simulink model "sim_line_seg_ctrl_with_pi_ctrl"  (R2021b)
settings: Solver=ode1  StartTime=0.0  StopTime=inf  FixedStep=0.01  RelTol=1e-3
libraries: slpidlib x2, mobileRoboticsLib x1
settings Model: Creator=ASUS  LastModifiedBy=ASUS

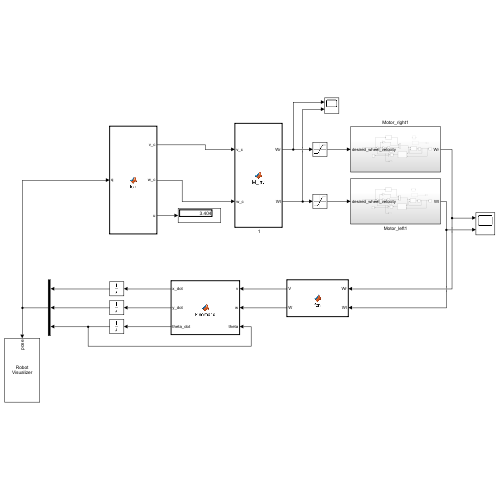
[thumbnail: Simulink's stored preview of the top-level diagram]
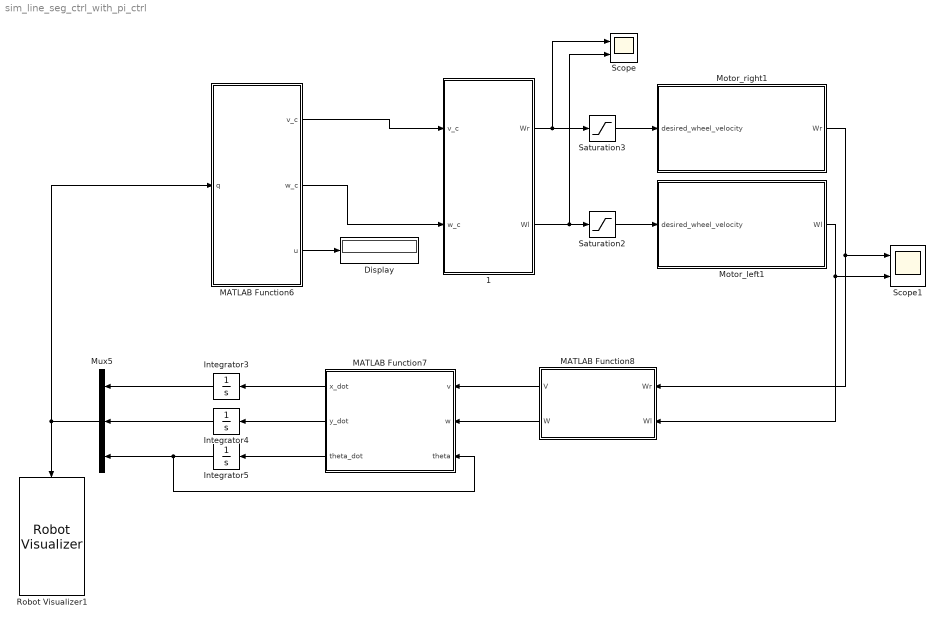
== system sim_line_seg_ctrl_with_pi_ctrl ==
  " 1" : MATLAB Function  TreatAsAtomicUnit=on
  Display : Display
  Integrator3 : Integrator  InitialCondition=5
  Integrator4 : Integrator  InitialCondition=1
  Integrator5 : Integrator  InitialCondition=0.6*pi
  MATLAB Function6 : MATLAB Function  TreatAsAtomicUnit=on
  MATLAB Function7 : MATLAB Function  TreatAsAtomicUnit=on
  MATLAB Function8 : MATLAB Function  TreatAsAtomicUnit=on
  Motor_left1 : Subsystem
  Motor_right1 : Subsystem
  Mux5 : Mux  Inputs=3
  Robot Visualizer1 : mobileRoboticsLib/Environments/Robot Visualizer  robotRadius=0.44  showTrajectory=on  hasWaypoints=off  hasLidar=off  sensorOffset=[ 0, 0 ]  scanAngles=[ -pi/4, 0, pi/4 ]  hasObjDetector=off  objDetectorOffset=[ 0, 0 ]  objDetectorAngle=0  objDetectorFOV=pi/4  objDetectorMaxRange=5  objectColors=[ 1, 0, 0; 0, 1, 0; 0, 0, 1 ]  objectMarkers=s
  Saturation2 : Saturate  UpperLimit=14  LowerLimit=-14
  Saturation3 : Saturate  UpperLimit=14  LowerLimit=-14
  Scope : Scope  NumInputPorts=2
  Scope1 : Scope  NumInputPorts=2
  wires:
  MATLAB Function7/2(y_dot) -> Integrator4/1
  Integrator5/1 -> Mux5/3, MATLAB Function7/3(theta)
  Integrator4/1 -> Mux5/2
  MATLAB Function8/1(V) -> MATLAB Function7/1(v)
  Integrator3/1 -> Mux5/1
  MATLAB Function8/2(W) -> MATLAB Function7/2(w)
  Mux5/1 -> Robot Visualizer1/1, MATLAB Function6/1(q)
  MATLAB Function7/1(x_dot) -> Integrator3/1
  MATLAB Function7/3(theta_dot) -> Integrator5/1
  MATLAB Function6/1(v_c) -> " 1"/1(v_c)
  MATLAB Function6/2(w_c) -> " 1"/2(w_c)
  " 1"/1(Wr) -> Scope/1, Saturation3/1
  Saturation3/1 -> Motor_right1/1(desired_wheel_velocity)
  " 1"/2(Wl) -> Scope/2, Saturation2/1
  Saturation2/1 -> Motor_left1/1(desired_wheel_velocity)
  Motor_right1/1(Wr) -> MATLAB Function8/1(Wr), Scope1/1
  Motor_left1/1(Wl) -> MATLAB Function8/2(Wl), Scope1/2
  MATLAB Function6/3(u) -> Display/1

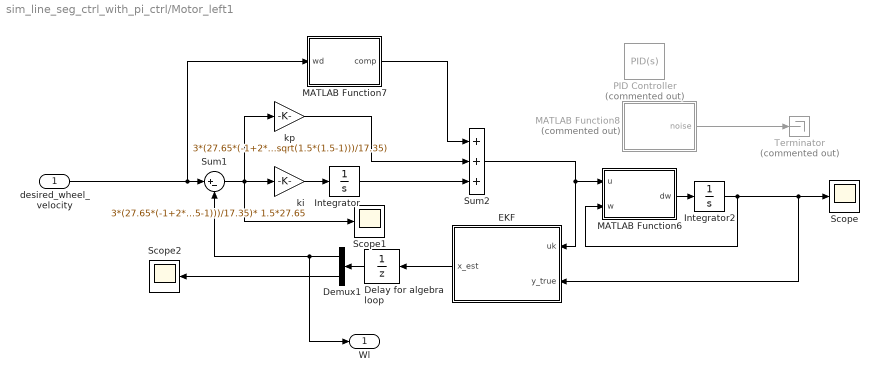
== system sim_line_seg_ctrl_with_pi_ctrl/Motor_left1 ==
  desired_wheel_velocity : Inport
  Delay for algebra loop : UnitDelay  SampleTime=-1  HasFrameUpgradeWarning=on
  Demux1 : Demux  Outputs=[1,3]
  EKF : MATLAB Function  TreatAsAtomicUnit=on
  Integrator : Integrator
  Integrator2 : Integrator
  MATLAB Function6 : MATLAB Function  TreatAsAtomicUnit=on
  MATLAB Function7 : MATLAB Function  TreatAsAtomicUnit=on
  MATLAB Function8 : MATLAB Function  Commented=on  TreatAsAtomicUnit=on
  PID Controller : slpidlib/PID Controller  Commented=on  Controller=PID  Form=Parallel  TimeDomain=Continuous-time  UseExternalTs=off  SampleTime=-1  IntegratorMethod=Forward Euler  FilterMethod=Forward Euler  ControllerParametersSource=internal  P=3*(27.65*(-1+2*1.5-2*sqrt(1.5*(1.5-1)))/17.35)  I=3*(27.65*(-1+2*1.5-2*sqrt(1.5*(1.5-1)))/17.35)* 1.5*27.65  D=0  UseFilter=on  N=100  TunerSelectOption=Transfer Function Based (PID Tuner App)  InitialConditionSource=internal  InitialConditionForIntegrator=0  InitialConditionForFilter=0  DifferentiatorICPrevScaledInput=0  ExternalReset=none  TrackingMode=off  Kt=1  LimitOutput=off  SatLimitsSource=internal  UpperSaturationLimit=inf  LowerSaturationLimit=-inf  LinearizeAsGain=on  AntiWindupMode=none  Kb=1  POutMin=[]  POutMax=[]  IOutMin=[]  IOutMax=[]  DOutMin=[]  DOutMax=[]  NOutMin=[]  NOutMax=[]  SumOutMin=[]  SumOutMax=[]  SaturationOutMin=[]  SaturationOutMax=[]  PParamMin=[]  PParamMax=[]  IParamMin=[]  IParamMax=[]  DParamMin=[]  DParamMax=[]  NParamMin=[]  NParamMax=[]  KbParamMin=[]  KbParamMax=[]  KtParamMin=[]  KtParamMax=[]  KbOutMin=[]  KbOutMax=[]  KtOutMin=[]  KtOutMax=[]  IntegratorOutMin=[]  IntegratorOutMax=[]  FilterOutMin=[]  FilterOutMax=[]  SumI1OutMin=[]  SumI1OutMax=[]  SumI2OutMin=[]  SumI2OutMax=[]  SumI3OutMin=[]  SumI3OutMax=[]  SumI4OutMin=[]  SumI4OutMax=[]  SumDOutMin=[]  SumDOutMax=[]  DifferentiatorOutMin=[]  DifferentiatorOutMax=[]  FilterDiffOutCoefMin=[]  FilterDiffOutCoefMax=[]  ReciprocalOutMin=[]  ReciprocalOutMax=[]  SumDenOutMin=[]  SumDenOutMax=[]  SumNumOutMin=[]  SumNumOutMax=[]  DivideOutMin=[]  DivideOutMax=[]  UdiffTsProdOutMin=[]  UdiffTsProdOutMax=[]  NTsProdOutMin=[]  NTsProdOutMax=[]  UintegralTsProdOutMin=[]  UintegralTsProdOutMax=[]  UngainTsProdOutMin=[]  UngainTsProdOutMax=[]  IntegratorContinuousStateAttributes=''  IntegratorStateMustResolveToSignalObject=off  IntegratorRTWStateStorageClass=Auto  FilterContinuousStateAttributes=''  FilterStateMustResolveToSignalObject=off  FilterRTWStateStorageClass=Auto  ParallelPVariant=InternalParameters  IdealPVariant=Disabled  IVariant=InternalParameters  DVariant=InternalParameters  IntegratorVariant=Continuous  SatVariant=Disabled  AWVariant=Passthrough  PCopyVariant=Disabled  TRVariant=Disabled  FdbkBlocksVariant=Forward  IdealPFdbkVariant=Disabled  SatFdbkVariant=Disabled  DerivativeFilterVariant=ContFilter  NVariant=InternalParameters  NCopyVariant=Disabled  FilterICVariant=InternalICsFilter  IntegratorICVariant=InternalICs  ExternalResetVariant=Disabled  TRSumVariant=Passthrough  SumFdbkVariant=Disabled  SumVariant=Sum_PID  TsampFilterVariant=InternalTs  TsampNgainVariant=Passthrough  TsampIntegralVariant=Passthrough  ExternalSaturationOutDataTypeStr=Inherit: Same as second input
  Scope : Scope
  Scope1 : Scope
  Scope2 : Scope
  Sum1 : Sum  Inputs=|+-
  Sum2 : Sum  Inputs=+++
  Terminator : Terminator  Commented=on
  ki : Gain  Gain=3*(27.65*(-1+2*1.5-2*sqrt(1.5*(1.5-1)))/17.35)* 1.5*27.65
  kp : Gain  Gain=3*(27.65*(-1+2*1.5-2*sqrt(1.5*(1.5-1)))/17.35)
  Wl : Outport
  wires:
  Sum2/1 -> MATLAB Function6/1(u), EKF/1(uk)
  MATLAB Function6/1(dw) -> Integrator2/1
  Integrator/1 -> Sum2/3
  kp/1 -> Sum2/2
  MATLAB Function7/1(comp) -> Sum2/1
  Demux1/1 -> Wl/1, Sum1/2
  Delay for algebra loop/1 -> Demux1/1
  desired_wheel_velocity/1 -> MATLAB Function7/1(wd), Sum1/1
  Sum1/1 -> ki/1, Scope1/1, kp/1
  ki/1 -> Integrator/1
  Demux1/2 -> Scope2/1
  MATLAB Function8/1(noise) -> Terminator/1
  Integrator2/1 -> MATLAB Function6/2(w), Scope/1, EKF/2(y_true)
  EKF/1(x_est) -> Delay for algebra loop/1

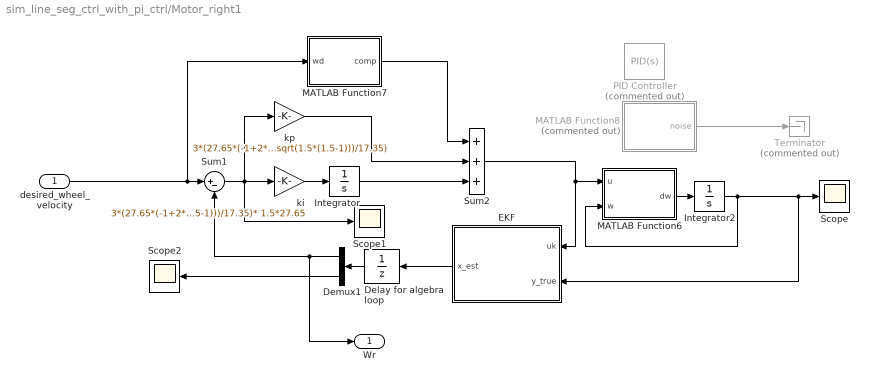
== system sim_line_seg_ctrl_with_pi_ctrl/Motor_right1 ==
  desired_wheel_velocity : Inport
  Delay for algebra loop : UnitDelay  SampleTime=-1  HasFrameUpgradeWarning=on
  Demux1 : Demux  Outputs=[1,3]
  EKF : MATLAB Function  TreatAsAtomicUnit=on
  Integrator : Integrator
  Integrator2 : Integrator
  MATLAB Function6 : MATLAB Function  TreatAsAtomicUnit=on
  MATLAB Function7 : MATLAB Function  TreatAsAtomicUnit=on
  MATLAB Function8 : MATLAB Function  Commented=on  TreatAsAtomicUnit=on
  PID Controller : slpidlib/PID Controller  Commented=on  Controller=PID  Form=Parallel  TimeDomain=Continuous-time  UseExternalTs=off  SampleTime=-1  IntegratorMethod=Forward Euler  FilterMethod=Forward Euler  ControllerParametersSource=internal  P=3*(27.65*(-1+2*1.5-2*sqrt(1.5*(1.5-1)))/17.35)  I=3*(27.65*(-1+2*1.5-2*sqrt(1.5*(1.5-1)))/17.35)* 1.5*27.65  D=0  UseFilter=on  N=100  TunerSelectOption=Transfer Function Based (PID Tuner App)  InitialConditionSource=internal  InitialConditionForIntegrator=0  InitialConditionForFilter=0  DifferentiatorICPrevScaledInput=0  ExternalReset=none  TrackingMode=off  Kt=1  LimitOutput=off  SatLimitsSource=internal  UpperSaturationLimit=inf  LowerSaturationLimit=-inf  LinearizeAsGain=on  AntiWindupMode=none  Kb=1  POutMin=[]  POutMax=[]  IOutMin=[]  IOutMax=[]  DOutMin=[]  DOutMax=[]  NOutMin=[]  NOutMax=[]  SumOutMin=[]  SumOutMax=[]  SaturationOutMin=[]  SaturationOutMax=[]  PParamMin=[]  PParamMax=[]  IParamMin=[]  IParamMax=[]  DParamMin=[]  DParamMax=[]  NParamMin=[]  NParamMax=[]  KbParamMin=[]  KbParamMax=[]  KtParamMin=[]  KtParamMax=[]  KbOutMin=[]  KbOutMax=[]  KtOutMin=[]  KtOutMax=[]  IntegratorOutMin=[]  IntegratorOutMax=[]  FilterOutMin=[]  FilterOutMax=[]  SumI1OutMin=[]  SumI1OutMax=[]  SumI2OutMin=[]  SumI2OutMax=[]  SumI3OutMin=[]  SumI3OutMax=[]  SumI4OutMin=[]  SumI4OutMax=[]  SumDOutMin=[]  SumDOutMax=[]  DifferentiatorOutMin=[]  DifferentiatorOutMax=[]  FilterDiffOutCoefMin=[]  FilterDiffOutCoefMax=[]  ReciprocalOutMin=[]  ReciprocalOutMax=[]  SumDenOutMin=[]  SumDenOutMax=[]  SumNumOutMin=[]  SumNumOutMax=[]  DivideOutMin=[]  DivideOutMax=[]  UdiffTsProdOutMin=[]  UdiffTsProdOutMax=[]  NTsProdOutMin=[]  NTsProdOutMax=[]  UintegralTsProdOutMin=[]  UintegralTsProdOutMax=[]  UngainTsProdOutMin=[]  UngainTsProdOutMax=[]  IntegratorContinuousStateAttributes=''  IntegratorStateMustResolveToSignalObject=off  IntegratorRTWStateStorageClass=Auto  FilterContinuousStateAttributes=''  FilterStateMustResolveToSignalObject=off  FilterRTWStateStorageClass=Auto  ParallelPVariant=InternalParameters  IdealPVariant=Disabled  IVariant=InternalParameters  DVariant=InternalParameters  IntegratorVariant=Continuous  SatVariant=Disabled  AWVariant=Passthrough  PCopyVariant=Disabled  TRVariant=Disabled  FdbkBlocksVariant=Forward  IdealPFdbkVariant=Disabled  SatFdbkVariant=Disabled  DerivativeFilterVariant=ContFilter  NVariant=InternalParameters  NCopyVariant=Disabled  FilterICVariant=InternalICsFilter  IntegratorICVariant=InternalICs  ExternalResetVariant=Disabled  TRSumVariant=Passthrough  SumFdbkVariant=Disabled  SumVariant=Sum_PID  TsampFilterVariant=InternalTs  TsampNgainVariant=Passthrough  TsampIntegralVariant=Passthrough  ExternalSaturationOutDataTypeStr=Inherit: Same as second input
  Scope : Scope
  Scope1 : Scope
  Scope2 : Scope
  Sum1 : Sum  Inputs=|+-
  Sum2 : Sum  Inputs=+++
  Terminator : Terminator  Commented=on
  ki : Gain  Gain=3*(27.65*(-1+2*1.5-2*sqrt(1.5*(1.5-1)))/17.35)* 1.5*27.65
  kp : Gain  Gain=3*(27.65*(-1+2*1.5-2*sqrt(1.5*(1.5-1)))/17.35)
  Wr : Outport
  wires:
  Sum2/1 -> MATLAB Function6/1(u), EKF/1(uk)
  desired_wheel_velocity/1 -> MATLAB Function7/1(wd), Sum1/1
  Sum1/1 -> ki/1, Scope1/1, kp/1
  kp/1 -> Sum2/2
  MATLAB Function6/1(dw) -> Integrator2/1
  EKF/1(x_est) -> Delay for algebra loop/1
  MATLAB Function8/1(noise) -> Terminator/1
  Demux1/2 -> Scope2/1
  MATLAB Function7/1(comp) -> Sum2/1
  Integrator2/1 -> MATLAB Function6/2(w), EKF/2(y_true), Scope/1
  Demux1/1 -> Wr/1, Sum1/2
  Delay for algebra loop/1 -> Demux1/1
  ki/1 -> Integrator/1
  Integrator/1 -> Sum2/3

== matlab function sim_line_seg_ctrl_with_pi_ctrl/Motor_right1/MATLAB Function7 ==
  settings: updateMethod=DISCRETE
  data: wd input; comp output
function comp = fcn(wd)

b = 17.35 + rand; c = 5.63 + 0.3*rand;
comp = c/b*sign(wd);

== matlab function sim_line_seg_ctrl_with_pi_ctrl/Motor_right1/MATLAB Function8 ==
  data: noise output
function noise = fcn

noise = 0.1*randn;

== matlab function sim_line_seg_ctrl_with_pi_ctrl/MATLAB Function6 ==
  settings: updateMethod=DISCRETE
  data: q input; v_c output; w_c output; u output
function [v_c,w_c,u] = fcn(q)

T = [3, 0; 6, 4; 3, 4; 3, 1; 0, 3].';

persistent i
if isempty(i)
    i = 1;
end

if i>4
    i = 4;
end

dx = T(1,i+1) - T(1,i);
dy = T(2,i+1) - T(2,i);

v = [dx; dy]; 
vN = [dy; -dx];
r = q(1:2) - T(:,i);
u = v.'*r/(v.'*v);
if u>1
    i = i+1;
end
dn = vN.'*r/(vN.'*vN); % Normalized orthogonal distance
phiLin = atan2(v(2), v(1));
phiRot = atan(5*dn);
phiRef = wrapToPi(phiLin + phiRot);

ePhi = wrapToPi(phiRef - q(3));

v_c = 0.8*cos(ePhi);
w_c = 3*ePhi;

== matlab function sim_line_seg_ctrl_with_pi_ctrl/ 1 ==
  data: v_c input; Wr output; w_c input; Wl output
function [Wr, Wl] = M_inv(v_c, w_c)
r = 0.07;      %wheel radius
b = 0.22;      %length from wheel to wheel

Wr = ((2*v_c)+(w_c*b))/(2*r);
Wl = ((2*v_c)-(w_c*b))/(2*r);

== matlab function sim_line_seg_ctrl_with_pi_ctrl/MATLAB Function7 ==
  data: v input; x_dot output; w input; y_dot output; theta_dot output; theta input
function [x_dot,y_dot,theta_dot]= kinematic(v,w,theta)
x_dot = v*cos(theta);
y_dot = v*sin(theta);
theta_dot = w;

== matlab function sim_line_seg_ctrl_with_pi_ctrl/MATLAB Function8 ==
  data: Wr input; V output; Wl input; W output
function [V,W]= fcn(Wr,Wl)
r = 0.07;      %wheel radius
b = 0.22;      %length from wheel to wheel

V = r*(Wr/2) + r*(Wl/2);
W = r*(Wr/b) - r*(Wl/b);

== matlab function sim_line_seg_ctrl_with_pi_ctrl/Motor_left1/EKF ==
  settings: updateMethod=DISCRETE
  data: uk input; y_true input; x_est output
function x_est = EKF(uk,y_true)
Ts=0.01;
persistent x_est_p P Qd_est R_est Qc_est;
if isempty(x_est_p)
    
    x_est_p=[2;13;25;1];
    P=2*eye(4);
    Qc_est=1e-5*diag([10,25,25,1]);
    Qd_est=Qc_est*Ts;
    R_est=0.02;
end
c=[1 0 0 0];D=0;Ck=c;Dk=D;
%Comput Kalman Gain and update predicted value
Wk=P*Ck'/(Ck*P*Ck'+R_est);
y_est=Ck*x_est_p+Dk*uk;
x=x_est_p+Wk.*(y_true-y_est);
%Compute prediction at next time step
x_est=x+Ts*[-x(2)*x(1)+uk*x(3)-x(4)*sign(x(1));0;0;0];
%Update error covariance matrices
P=P-Wk*Ck*P;
%Define Ak
Ak=eye(4)+Ts*[-x(2) -x(1) uk -sign(x(1));0 0 0 0;0 0 0 0;0 0 0 0]; % jacobian
P=Ak*P*Ak'+Qd_est;
x_est_p=x_est;

== matlab function sim_line_seg_ctrl_with_pi_ctrl/Motor_left1/MATLAB Function6 ==
  settings: updateMethod=DISCRETE
  data: u input; dw output; w input
function dw = dcmotor(u,w)

a = 27.65; b = 17.35; c = 5.63;
dw = -a*w+b*u-c*sign(w) + 1e-4*randn;

== matlab function sim_line_seg_ctrl_with_pi_ctrl/Motor_left1/MATLAB Function7 ==
  settings: updateMethod=DISCRETE
  data: wd input; comp output
function comp = fcn(wd)

b = 17.35 + rand; c = 5.63 + 0.3*rand;
comp = c/b*sign(wd);

== matlab function sim_line_seg_ctrl_with_pi_ctrl/Motor_left1/MATLAB Function8 ==
  data: noise output
function noise = fcn

noise = 0.1*randn;

== matlab function sim_line_seg_ctrl_with_pi_ctrl/Motor_right1/EKF ==
  settings: updateMethod=DISCRETE
  data: uk input; y_true input; x_est output
function x_est = EKF(uk,y_true)
Ts=0.01;
persistent x_est_p P Qd_est R_est Qc_est;
if isempty(x_est_p)
    
    x_est_p=[2;13;25;1];
    P=2*eye(4);
    Qc_est=1e-5*diag([10,25,25,1]);
    Qd_est=Qc_est*Ts;
    R_est=0.02;
end
c=[1 0 0 0];D=0;Ck=c;Dk=D;
%Comput Kalman Gain and update predicted value
Wk=P*Ck'/(Ck*P*Ck'+R_est);
y_est=Ck*x_est_p+Dk*uk;
x=x_est_p+Wk.*(y_true-y_est);
%Compute prediction at next time step
x_est=x+Ts*[-x(2)*x(1)+uk*x(3)-x(4)*sign(x(1));0;0;0];
%Update error covariance matrices
P=P-Wk*Ck*P;
%Define Ak
Ak=eye(4)+Ts*[-x(2) -x(1) uk -sign(x(1));0 0 0 0;0 0 0 0;0 0 0 0]; % jacobian
P=Ak*P*Ak'+Qd_est;
x_est_p=x_est;

== matlab function sim_line_seg_ctrl_with_pi_ctrl/Motor_right1/MATLAB Function6 ==
  settings: updateMethod=DISCRETE
  data: u input; dw output; w input
function dw = dcmotor(u,w)

a = 27.65; b = 17.35; c = 5.63;
dw = -a*w+b*u-c*sign(w) + 1e-4*randn;
